simulink model "PositionControl"  (R2019b)
settings: Solver=ode3  StartTime=0.0  StopTime=100.0  FixedStep=Ts  RelTol=1e-3
values from neighbouring files (symbols this model uses):
  refx = 2.0    (= 2)    [RunPositionControl_b.m]    (also in RunPositionControl_d.m; RunPositionControl_e.m = 10 * rand - 5; RunPositionControl_i.m = 10 * rand - 5)
  refy = 2.0    (= 2)    [RunPositionControl_b.m]    (also in RunPositionControl_d.m; RunPositionControl_e.m = 10 * rand - 5; RunPositionControl_i.m = 10 * rand - 5)
undefined symbols (not defined in the file or in its folder): DiscIntNeverNeededParam
libraries: simulink x1
settings Model: Creator=Pablo  LastModifiedBy=Pablo
settings DataIOCC: ReturnWorkspaceOutputs=off

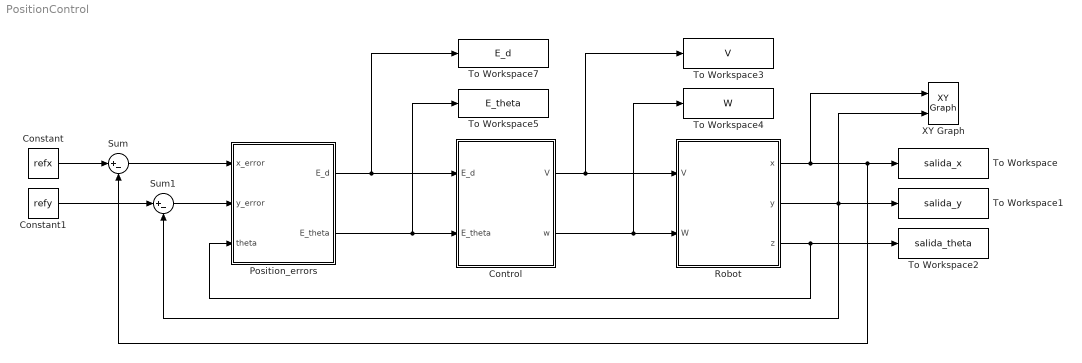
== system PositionControl ==
  Constant : Constant  Value=refx
  Constant1 : Constant  Value=refy
  Control : Subsystem
  Position_errors : Subsystem
  "Robot " : Subsystem
  Sum : Sum  Inputs=|+-
  Sum1 : Sum  Inputs=|+-
  To Workspace : ToWorkspace  VariableName=salida_x  SaveFormat=Structure With Time  SampleTime=-1
  To Workspace1 : ToWorkspace  VariableName=salida_y  SaveFormat=Structure With Time  SampleTime=-1
  To Workspace2 : ToWorkspace  VariableName=salida_theta  SaveFormat=Structure With Time  SampleTime=-1
  To Workspace3 : ToWorkspace  VariableName=V  SaveFormat=Structure With Time  SampleTime=-1
  To Workspace4 : ToWorkspace  VariableName=W  SaveFormat=Structure With Time  SampleTime=-1
  To Workspace5 : ToWorkspace  VariableName=E_theta  SaveFormat=Structure With Time  SampleTime=-1
      settings: Save2DSignal=2-D array (concatenate along first dimension)
  To Workspace7 : ToWorkspace  VariableName=E_d  SaveFormat=Structure With Time  SampleTime=-1
      settings: Save2DSignal=2-D array (concatenate along first dimension)
  XY Graph : simulink/Sinks/XY Graph  xmin=-5  xmax=5  ymin=-5  ymax=5  st=-1
  wires:
  Control/1(V) -> "Robot "/1("V "), To Workspace3/1
  Control/2(w) -> "Robot "/2("W "), To Workspace4/1
  "Robot "/3(z) -> Position_errors/3(theta), To Workspace2/1
  "Robot "/2(y) -> To Workspace1/1, XY Graph/2, Sum1/2
  "Robot "/1(x) -> XY Graph/1, To Workspace/1, Sum/2
  Constant/1 -> Sum/1
  Constant1/1 -> Sum1/1
  Position_errors/2(E_theta) -> To Workspace5/1, Control/2(E_theta)
  Sum1/1 -> Position_errors/2(y_error)
  Sum/1 -> Position_errors/1(x_error)
  Position_errors/1(E_d) -> To Workspace7/1, Control/1(E_d)

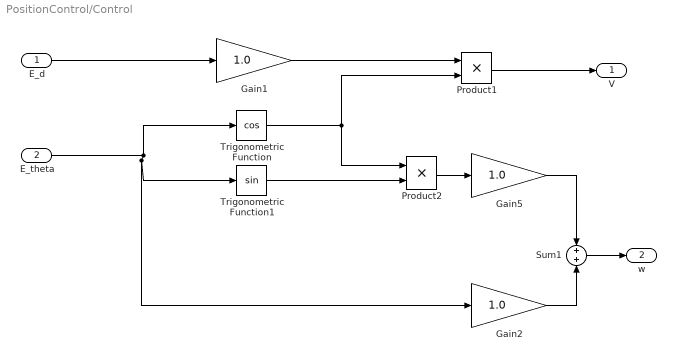
== system PositionControl/Control ==
  E_d : Inport
  E_theta : Inport  Port=2
  Gain1 : Gain  Gain=1.0
  Gain2 : Gain  Gain=1.0
  Gain5 : Gain  Gain=1.0
  Product1 : Product
  Product2 : Product
  Sum1 : Sum
  Trigonometric Function : Trigonometry  Operator=cos
  Trigonometric Function1 : Trigonometry
  V : Outport  VectorParamsAs1DForOutWhenUnconnected=off
  w : Outport  Port=2  VectorParamsAs1DForOutWhenUnconnected=off
  wires:
  E_theta/1 -> Trigonometric Function/1, Trigonometric Function1/1, Gain2/1
  E_d/1 -> Gain1/1
  Trigonometric Function/1 -> Product1/2, Product2/1
  Product1/1 -> V/1
  Trigonometric Function1/1 -> Product2/2
  Product2/1 -> Gain5/1
  Gain1/1 -> Product1/1
  Gain5/1 -> Sum1/1
  Gain2/1 -> Sum1/2
  Sum1/1 -> w/1

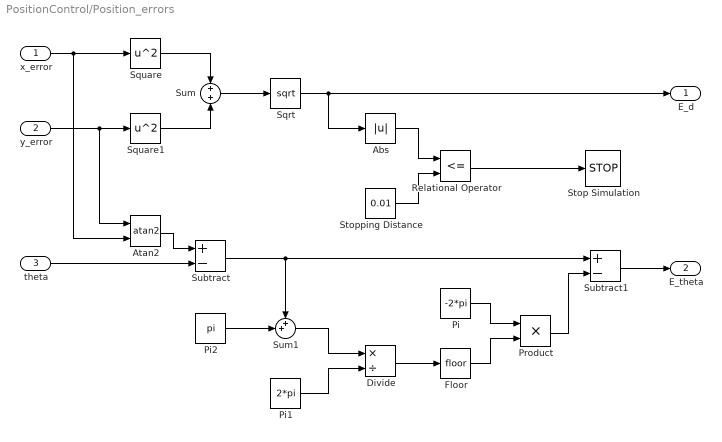
== system PositionControl/Position_errors ==
  x_error : Inport
  y_error : Inport  Port=2
  theta : Inport  Port=3
  Abs : Abs
  Atan2 : Trigonometry  Operator=atan2
  Divide : Product  Inputs=*/
  Floor : Rounding
  Pi : Constant  Value=-2*pi  OutDataTypeStr=Inherit: Inherit via back propagation
  Pi1 : Constant  Value=2*pi  OutDataTypeStr=Inherit: Inherit via back propagation
  Pi2 : Constant  Value=pi  OutDataTypeStr=Inherit: Inherit via back propagation
  Product : Product
  Relational Operator : RelationalOperator  Operator=<=  OutDataTypeStr=boolean  RndMeth=Simplest
  Sqrt : Sqrt  SaturateOnIntegerOverflow=on
  Square : Math  Operator=square  SignedPower=off  SaturateOnIntegerOverflow=on
  Square1 : Math  Operator=square  SignedPower=off  SaturateOnIntegerOverflow=on
  "Stop Simulation " : Stop
  Stopping Distance : Constant  Value=0.01
  Subtract : Sum  Inputs=+-
  Subtract1 : Sum  Inputs=+-
  Sum : Sum  Inputs=+|+
  Sum1 : Sum  Inputs=++|
  E_d : Outport
  E_theta : Outport  Port=2
  wires:
  y_error/1 -> Atan2/1, Square1/1
  x_error/1 -> Atan2/2, Square/1
  Sqrt/1 -> E_d/1, Abs/1
  Relational Operator/1 -> "Stop Simulation "/1
  Sum1/1 -> Divide/1
  Product/1 -> Subtract1/2
  theta/1 -> Subtract/2
  Pi1/1 -> Divide/2
  Sum/1 -> Sqrt/1
  Atan2/1 -> Subtract/1
  Subtract/1 -> Subtract1/1, Sum1/1
  Divide/1 -> Floor/1
  Pi/1 -> Product/1
  Subtract1/1 -> E_theta/1
  Abs/1 -> Relational Operator/1
  Floor/1 -> Product/2
  Stopping Distance/1 -> Relational Operator/2
  Pi2/1 -> Sum1/2
  Square/1 -> Sum/1
  Square1/1 -> Sum/2

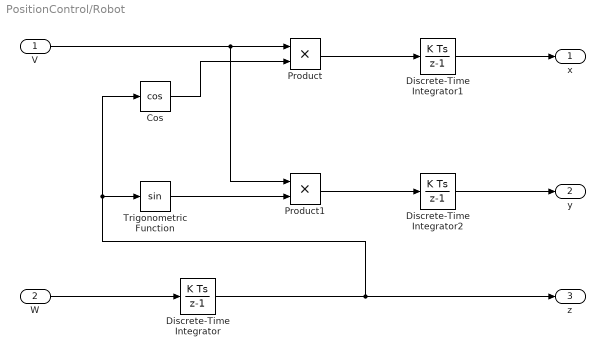
== system PositionControl/Robot  ==
  "V " : Inport
  "W " : Inport  Port=2
  Cos : Trigonometry  Operator=cos
  Discrete-Time Integrator : DiscreteIntegrator  SampleTime=-1  ICPrevOutput=DiscIntNeverNeededParam  ICPrevScaledInput=DiscIntNeverNeededParam
  Discrete-Time Integrator1 : DiscreteIntegrator  SampleTime=-1  ICPrevOutput=DiscIntNeverNeededParam  ICPrevScaledInput=DiscIntNeverNeededParam
  Discrete-Time Integrator2 : DiscreteIntegrator  SampleTime=-1  ICPrevOutput=DiscIntNeverNeededParam  ICPrevScaledInput=DiscIntNeverNeededParam
  Product : Product
  Product1 : Product
  Trigonometric Function : Trigonometry
  x : Outport
  y : Outport  Port=2
  z : Outport  Port=3
  wires:
  Product/1 -> Discrete-Time Integrator1/1
  Trigonometric Function/1 -> Product1/2
  Discrete-Time Integrator/1 -> z/1, Cos/1, Trigonometric Function/1
  "W "/1 -> Discrete-Time Integrator/1
  Product1/1 -> Discrete-Time Integrator2/1
  Cos/1 -> Product/2
  "V "/1 -> Product1/1, Product/1
  Discrete-Time Integrator2/1 -> y/1
  Discrete-Time Integrator1/1 -> x/1
